simulink model "Models"  (Simulink 8.0)
settings: Solver=ode45  StartTime=0.0  StopTime=10.0  RelTol=1e-3
settings Model: Creator=Faradars  LastModifiedBy=Faradars

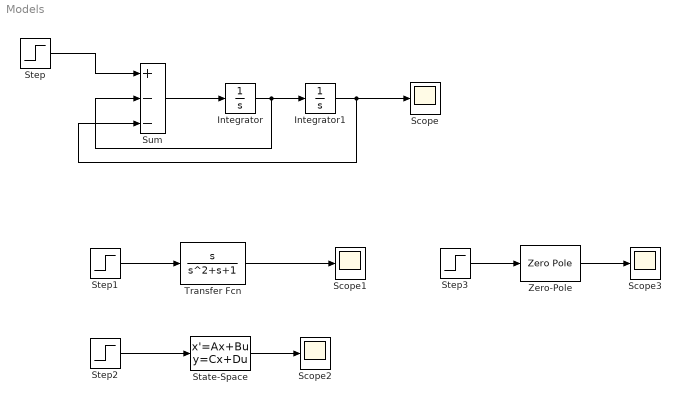
== system Models ==
  Integrator : Integrator
  Integrator1 : Integrator
  Scope{,1..3} (4 alike) : Scope
      Scope2 settings: SaveName=ScopeData2
      Scope3 settings: SaveName=ScopeData3
  State-Space : StateSpace  A=[0 1; -1 -1]  B=[0; 1]  C=[0 1]  D=0
  Step{,1..3} (4 alike) : Step  Before=0.1  SampleTime=15
  Sum : Sum  Inputs=+--
  Transfer Fcn : TransferFcn  Numerator=[1 0]  Denominator=[1 1 1]
  Zero-Pole : ZeroPole  Zeros=[0]  Poles=[1 -1]  Gain=[4]
  wires:
  Sum/1 -> Integrator/1
  Integrator/1 -> Sum/2, Integrator1/1
  Integrator1/1 -> Sum/3, Scope/1
  Step/1 -> Sum/1
  Transfer Fcn/1 -> Scope1/1
  Step1/1 -> Transfer Fcn/1
  State-Space/1 -> Scope2/1
  Step2/1 -> State-Space/1
  Zero-Pole/1 -> Scope3/1
  Step3/1 -> Zero-Pole/1
